simulink model "fuzzy"  (R2018b)
settings: Solver=VariableStepAuto  StartTime=0.0  StopTime=10.0  RelTol=1e-3
libraries: fuzblock x1
settings Model: Creator=student  LastModifiedBy=student

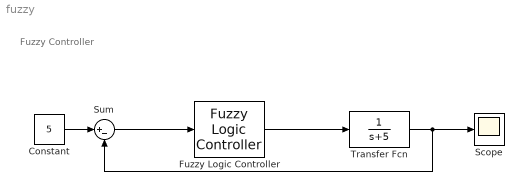
== system fuzzy ==
  note: Fuzzy Controller
  Constant : Constant  Value=5
  Fuzzy Logic Controller : fuzblock/Fuzzy Logic  Controller  FIS='xyz3013.fis'  OutputSampleNumber=101  DataType=double  FuzzifiedInputs=off  RuleFiringStrengths=off  RuleOutputs=off  AggregatedOutputs=off  SimulateUsing=Interpreted execution  OutOfRangeInputValueMessage=warning  NoRuleFiredMessage=warning  EmptyOutputFuzzySetMessage=warning
  Scope : Scope
  Sum : Sum  Inputs=|+-
  Transfer Fcn : TransferFcn  Denominator=[1 5]
  wires:
  Sum/1 -> Fuzzy Logic Controller/1
  Fuzzy Logic Controller/1 -> Transfer Fcn/1
  Transfer Fcn/1 -> Sum/2, Scope/1
  Constant/1 -> Sum/1
